simulink model "flight_simulation"  (R2021b)
settings: Solver=VariableStepAuto  StartTime=0.0  StopTime=50  RelTol=1e-3
undefined symbols (not defined in the file or in its folder): Earth, WGS84
libraries: dspsrcs4 x3, aerolibfltsims x2, aerolibtransform2 x1
settings Model: Creator=LENOVO  LastModifiedBy=LENOVO

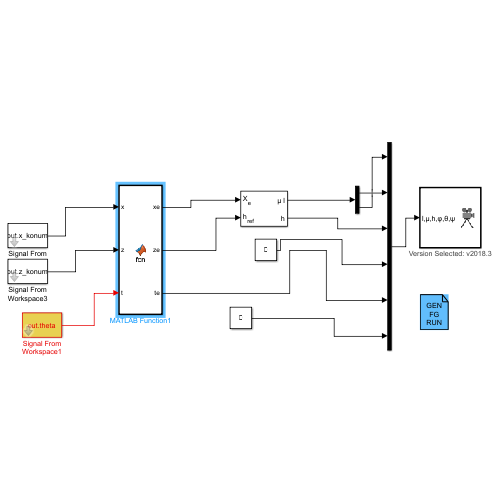
[thumbnail: Simulink's stored preview of the top-level diagram]
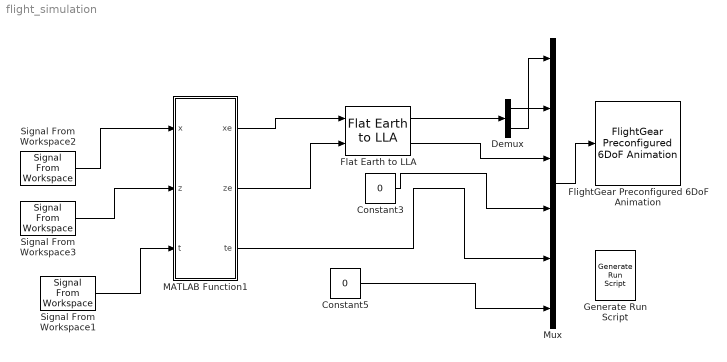
== system flight_simulation ==
  Constant3 : Constant  Value=0
  Constant5 : Constant  Value=0
  Demux : Demux  Outputs=2
  Flat Earth to LLA : aerolibtransform2/Flat Earth to LLA  units=Metric (MKS)  ptype=Earth (WGS84)  F=1/298.257223563  R=6378137  refPosPort=off  LL0=[0 10]  psi=0
  FlightGear Preconfigured 6DoF Animation : aerolibfltsims/FlightGear Preconfigured 6DoF Animation  xFlightGearVersion=v2018.3  DestinationIpAddress=127.0.0.1  DestinationPort=5502  SampleTime=1/30  packetVersion=24
  Generate Run Script : aerolibfltsims/Generate Run Script  Architecture=Win64  dataFlow=Send  GeometryModelName=milal  AirportId=KSFO  RunwayId=10L  InitialAltitude=7224  InitialHeading=113  OffsetDistance=4.72  OffsetAzimuth=0  InstallScenery=on  DisableShaders=off  OriginAddress=127.0.0.1  DestinationPort=5502  OriginPort=5505  LocalAddress=127.0.0.1  OutputFileName=runfg.bat  FlightGearBaseDirectory=C:\Program Files\FlightGear 2020.3
  MATLAB Function1 : MATLAB Function  TreatAsAtomicUnit=on
  Mux : Mux  Inputs=6
  Signal From Workspace1 : dspsrcs4/Signal From Workspace  X=out.theta  Ts=0.1  nsamps=1  OutputAfterFinalValue=Setting to zero  ignoreOrWarnInputAndFrameLengths=off  OutputFrames=off
  Signal From Workspace2 : dspsrcs4/Signal From Workspace  X=out.x_konum  Ts=0.1  nsamps=1  OutputAfterFinalValue=Setting to zero  ignoreOrWarnInputAndFrameLengths=off  OutputFrames=off
  Signal From Workspace3 : dspsrcs4/Signal From Workspace  X=out.z_konum  Ts=0.1  nsamps=1  OutputAfterFinalValue=Setting to zero  ignoreOrWarnInputAndFrameLengths=off  OutputFrames=off
  wires:
  Signal From Workspace1/1 -> MATLAB Function1/3(t)
  MATLAB Function1/3(te) -> Mux/5
  Signal From Workspace3/1 -> MATLAB Function1/2(z)
  Demux/2 -> Mux/1
  MATLAB Function1/1(xe) -> Flat Earth to LLA/1
  Flat Earth to LLA/2 -> Mux/3
  Mux/1 -> FlightGear Preconfigured 6DoF Animation/1
  Constant3/1 -> Mux/4
  Constant5/1 -> Mux/6
  Signal From Workspace2/1 -> MATLAB Function1/1(x)
  Demux/1 -> Mux/2
  Flat Earth to LLA/1 -> Demux/1
  MATLAB Function1/2(ze) -> Flat Earth to LLA/2

== matlab function flight_simulation/MATLAB Function1 ==
  data: x input; xe output; z input; ze output; te output; t input
function [xe,ze,te] = fcn(x,z,t)
te=t(1,1)/8+pi;
xe=-[x(1,1)*2 ;0 ; 0];
ze=-(z(1,1)+15);
end
